simulink model "OBM_repeat"  (R2020a)
settings: Solver=FixedStepAuto  StartTime=186*86400  StopTime=191*86400  FixedStep=60  RelTol=1e-3
settings Model: Creator=zhelu  LastModifiedBy=yl3328

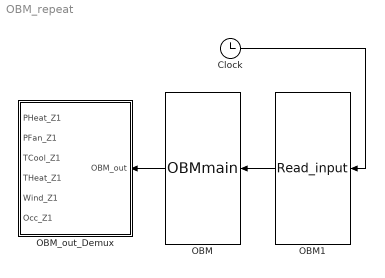
== system OBM_repeat ==
  Clock : Clock
  OBM : M-S-Function  FunctionName=OBMmain
  OBM1 : M-S-Function  FunctionName=Read_input
  OBM_out_Demux : MATLAB Function  TreatAsAtomicUnit=on
  wires:
  OBM/1 -> OBM_out_Demux/1(OBM_out)
  OBM1/1 -> OBM/1
  Clock/1 -> OBM1/1

== matlab function OBM_repeat/OBM_out_Demux ==
  data: OBM_out input; PHeat_Z1 output; PFan_Z1 output; TCool_Z1 output; THeat_Z1 output; Wind_Z1 output; Occ_Z1 output
function [PHeat_Z1,PFan_Z1,TCool_Z1,THeat_Z1,Wind_Z1,Occ_Z1] = fcn(OBM_out)

PHeat_Z1 = OBM_out(1);
PFan_Z1 = OBM_out(2);
TCool_Z1 = OBM_out(3);
THeat_Z1 = OBM_out(4);
Wind_Z1 = OBM_out(5);
Occ_Z1 = OBM_out(6);
